simulink model "ex13"  (Simulink 6.3)
settings: Solver=VariableStepDiscrete  StartTime=0.0  StopTime=10  RelTol=1e-3
undefined symbols (not defined in the file or in its folder): gfprimfd
libraries: dspbuff3 x5, commblkcod2 x3, commsink2 x2, commblkintrlv2 x2, commnoisgen2 x1, commrandsrc2 x1
settings Model: LastModifiedBy=lxy  StrictBusMsg=None
settings OptimizationCC: InlineInvariantSignals=on

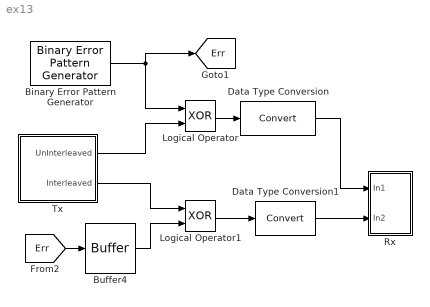
== system ex13 ==
  Binary Error Pattern Generator : commnoisgen2/Binary Error Pattern Generator  n=15  prob=0.001*ones(1,8)  seed=12345  Ts=1/150000  frameBased=on  blksPerFrame=1  orient=off
  Buffer4 : dspbuff3/Buffer  N=30*20  V=0  ic=0
  Data Type Conversion : DataTypeConversion  OutDataTypeMode=double
  Data Type Conversion1 : DataTypeConversion  OutDataTypeMode=double
  Logical Operator : Logic  Operator=XOR  AllPortsSameDT=off  OutDataTypeMode=Boolean
  Logical Operator1 : Logic  Operator=XOR  AllPortsSameDT=off  OutDataTypeMode=Boolean  LogicDataType=double
  Rx : Subsystem
  Tx : Subsystem
  tag scope: Err=global
  wires:
  Logical Operator/1 -> Data Type Conversion/1
  Data Type Conversion/1 -> Rx/1(In1)
  [Err] -> Buffer4/1
  Tx/2(Interleaved) -> Logical Operator1/1
  Buffer4/1 -> Logical Operator1/2
  Data Type Conversion1/1 -> Rx/2(In2)
  Logical Operator1/1 -> Data Type Conversion1/1
  Binary Error Pattern Generator/1 -> [Err], Logical Operator/1
  Tx/1(UnInterleaved) -> Logical Operator/2

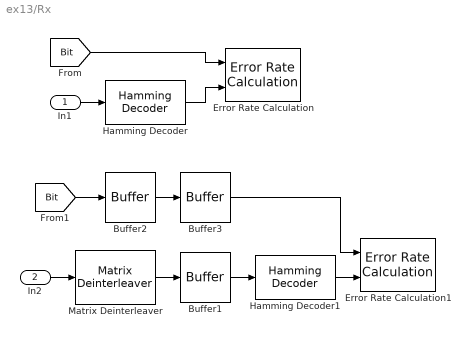
== system ex13/Rx ==
  In1 : Inport
  In2 : Inport  Port=2
  Buffer1 : dspbuff3/Buffer  N=15  V=0  ic=0
  Buffer2 : dspbuff3/Buffer  N=440  V=0  ic=0
  Buffer3 : dspbuff3/Buffer  N=11  V=0  ic=0
  Error Rate Calculation : commsink2/Error Rate Calculation  N=0  st_delay=0  cp_mode=Entire frame  subframe=[]  PMode=Workspace  WsName=BER2  RsMode2=off  stop=off  numErr=100  maxBits=1e6
  Error Rate Calculation1 : commsink2/Error Rate Calculation  N=0  st_delay=440  cp_mode=Entire frame  subframe=[]  PMode=Workspace  WsName=BER1  RsMode2=off  stop=off  numErr=100  maxBits=1e6
  Hamming Decoder : commblkcod2/Hamming Decoder  n=15  k=gfprimfd(4,'min')
  Hamming Decoder1 : commblkcod2/Hamming Decoder  n=15  k=gfprimfd(4,'min')
  Matrix Deinterleaver : commblkintrlv2/Matrix Deinterleaver  Nrows=30  Ncols=20
  wires:
  Hamming Decoder/1 -> Error Rate Calculation/2
  Matrix Deinterleaver/1 -> Buffer1/1
  Hamming Decoder1/1 -> Error Rate Calculation1/2
  [Bit] -> Error Rate Calculation/1
  [Bit] -> Buffer2/1
  Buffer2/1 -> Buffer3/1
  In1/1 -> Hamming Decoder/1
  In2/1 -> Matrix Deinterleaver/1
  Buffer3/1 -> Error Rate Calculation1/1
  Buffer1/1 -> Hamming Decoder1/1

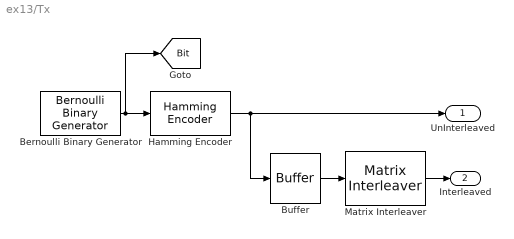
== system ex13/Tx ==
  Bernoulli Binary Generator : commrandsrc2/Bernoulli Binary Generator  P=0.5  seed=61  Ts=1/110000  frameBased=on  sampPerFrame=11  orient=off  outDataType=double
  Buffer : dspbuff3/Buffer  N=30*20  V=0  ic=0
  Hamming Encoder : commblkcod2/Hamming Encoder  n=15  k=gfprimfd(4,'min')
  Matrix Interleaver : commblkintrlv2/Matrix Interleaver  Nrows=30  Ncols=20
  UnInterleaved : Outport
  Interleaved : Outport  Port=2
  tag scope: Bit=global
  wires:
  Bernoulli Binary Generator/1 -> Hamming Encoder/1, [Bit]
  Hamming Encoder/1 -> Buffer/1, UnInterleaved/1
  Buffer/1 -> Matrix Interleaver/1
  Matrix Interleaver/1 -> Interleaved/1
